simulink model "tcp_aqm_fluid_flow"  (R2013a)
settings: Solver=ode45  StartTime=0.0  StopTime=10.0  RelTol=1e-3
undefined symbols (not defined in the file): N, R
settings Model: Creator=tohoanglinh  LastModifiedBy=tohoanglinh

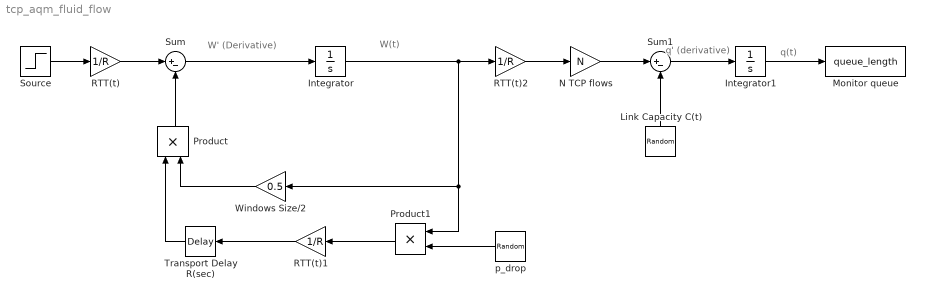
== system tcp_aqm_fluid_flow ==
  note: q(t)
  note: q' (derivative)
  note: W(t)
  note: W' (Derivative)
  Integrator : Integrator
  Integrator1 : Integrator
  Link Capacity C(t) : RandomNumber  SampleTime=0.1
  Monitor queue : ToWorkspace  VariableName=queue_length  SampleTime=-1  SaveFormat=Timeseries
  N TCP flows : Gain  Gain=N
  Product : Product
  Product1 : Product
  RTT(t) : Gain  Gain=1/R
  RTT(t)1 : Gain  Gain=1/R
  RTT(t)2 : Gain  Gain=1/R
  Source : Step  SampleTime=0
  Sum : Sum  Inputs=|+-
  Sum1 : Sum  Inputs=|+-
  Transport Delay R(sec) : TransportDelay
  Windows Size/2 : Gain  Gain=0.5
  p_drop : RandomNumber  SampleTime=0.1
  wires:
  Source/1 -> RTT(t)/1
  RTT(t)/1 -> Sum/1
  Product/1 -> Sum/2
  Windows Size/2/1 -> Product/2
  RTT(t)1/1 -> Transport Delay R(sec)/1
  Transport Delay R(sec)/1 -> Product/1
  Product1/1 -> RTT(t)1/1
  p_drop/1 -> Product1/2
  RTT(t)2/1 -> N TCP flows/1
  Sum/1 -> Integrator/1
  Integrator/1 -> Product1/1, Windows Size/2/1, RTT(t)2/1
  N TCP flows/1 -> Sum1/1
  Sum1/1 -> Integrator1/1
  Link Capacity C(t)/1 -> Sum1/2
  Integrator1/1 -> Monitor queue/1
